simulink library "trot_Gait"  (R2024a)
settings: Solver=VariableStepAuto  StartTime=0.0  StopTime=10.0  RelTol=1e-3
undefined symbols (not defined in the file): Lower_limbs, P0x, P0z, P1x, P1z, P2x, P2z, P3x, P3z, Upper_limbs
libraries: Plane_Movement_trot_forward x4
settings Model: Creator=renre  LastModifiedBy=renre

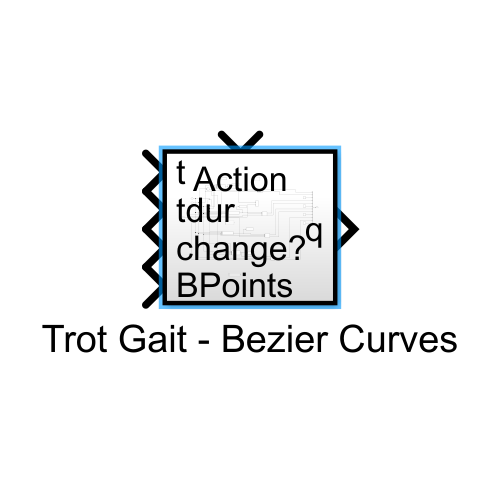
[thumbnail: Simulink's stored preview of the top-level diagram]
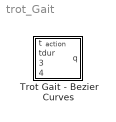
== system trot_Gait ==
  Trot Gait - Bezier Curves : Subsystem

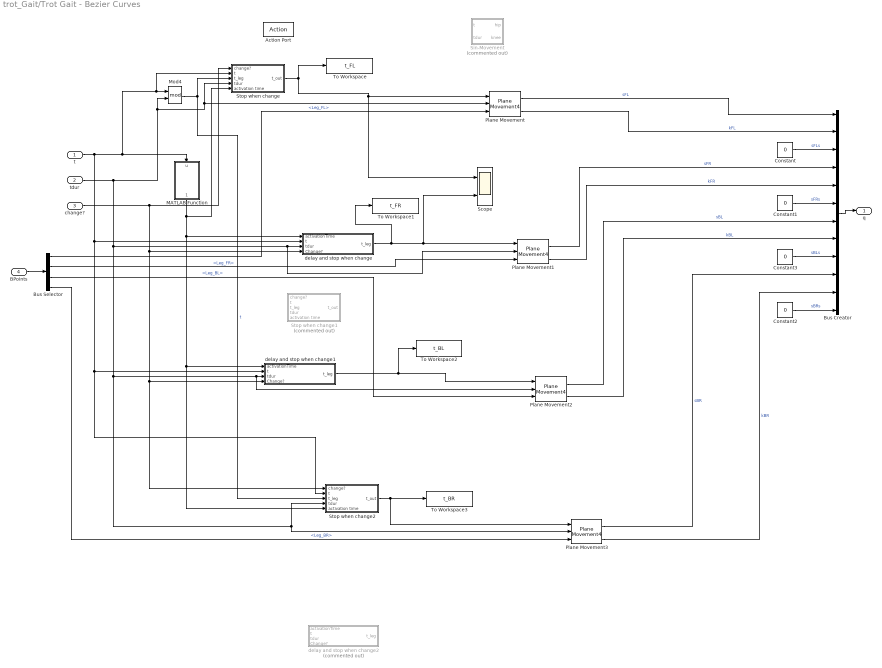
== system trot_Gait/Trot Gait - Bezier Curves ==
  t : Inport
  tdur : Inport  Port=2
  change? : Inport  Port=3
  BPoints : Inport  Port=4
  Action Port : ActionPort  InitializeStates=reset
  Bus Creator : BusCreator  Inputs=12
  Bus Selector : BusSelector  OutputSignals=Leg_FL,Leg_FR,Leg_BL,Leg_BR
  Constant{,1..3} (4 alike) : Constant  Value=0
  MATLAB Function : MATLAB Function  TreatAsAtomicUnit=on
  Mod4 : Math  Operator=mod
  Plane Movement{,1..3} (4 alike) : Plane_Movement_trot_forward/Plane Movement4  SystemSampleTime=-1  VariantActivationTime=update diagram  AllowFlexibleInterface=on  Latency=0  AutoFrameSizeCalculation=off
  Scope : Scope  NumInputPorts=2
  Sin-Movement : Subsystem  Commented=on
  Stop when change : Subsystem
  Stop when change1 : Subsystem  Commented=on
  Stop when change2 : Subsystem
  To Workspace : ToWorkspace  VariableName=t_FL  SaveFormat=Structure With Time  SampleTime=-1
  To Workspace1 : ToWorkspace  VariableName=t_FR  SaveFormat=Structure  SampleTime=-1
  To Workspace2 : ToWorkspace  VariableName=t_BL  SaveFormat=Structure  SampleTime=-1
  To Workspace3 : ToWorkspace  VariableName=t_BR  SaveFormat=Structure  SampleTime=-1
  delay and stop when change : Subsystem  mask{delay=0.5}
  delay and stop when change1 : Subsystem  mask{delay=0.5}
  delay and stop when change2 : Subsystem  Commented=on  mask{delay=0}
  q : Outport
  wires:
  BPoints/1 -> Bus Selector/1
  Stop when change/1(t_out) -> To Workspace/1, Plane Movement/1, Scope/1
  Stop when change2/1(t_out) -> Plane Movement3/1, To Workspace3/1
  delay and stop when change1/1(t_leg) -> Plane Movement2/1, To Workspace2/1
  delay and stop when change/1(t_leg) -> Plane Movement1/1, Scope/2, To Workspace1/1
  MATLAB Function/1(activationTime) -> delay and stop when change/1(activationTime), delay and stop when change1/1(activationTime), Stop when change2/5(activation time), Stop when change/5(activation time)
  change?/1 -> delay and stop when change/4(Change?), delay and stop when change1/4(Change?), Stop when change2/1(change?), Stop when change/1(change?)
  Constant2/1 -> Bus Creator/12  "sBRs"
  Constant3/1 -> Bus Creator/9  "sBLs"
  Constant1/1 -> Bus Creator/6  "sFRs"
  Constant/1 -> Bus Creator/3  "sFLs"
  Mod4/1 -> Stop when change/3(t_leg), Stop when change2/3(t_leg)  "t"
  tdur/1 -> delay and stop when change1/3(tdur), Plane Movement2/2, Plane Movement3/2, Stop when change2/4(tdur), delay and stop when change/3(tdur), Plane Movement1/2, Mod4/2, Plane Movement/2, Stop when change/4(tdur)
  t/1 -> Mod4/1, Stop when change/2(t), MATLAB Function/1(u), delay and stop when change/2(t), delay and stop when change1/2(t), Stop when change2/2(t)
  Plane Movement3/1 -> Bus Creator/10  "sBR"
  Plane Movement3/2 -> Bus Creator/11  "kBR"
  Plane Movement2/1 -> Bus Creator/7  "sBL"
  Plane Movement2/2 -> Bus Creator/8  "kBL"
  Plane Movement1/2 -> Bus Creator/5  "kFR"
  Plane Movement/2 -> Bus Creator/2  "kFL"
  Plane Movement1/1 -> Bus Creator/4  "sFR"
  Plane Movement/1 -> Bus Creator/1  "sFL"
  Bus Creator/1 -> q/1
  Bus Selector/1 -> Plane Movement/3  "<Leg_FL>"
  Bus Selector/2 -> Plane Movement1/3  "<Leg_FR>"
  Bus Selector/3 -> Plane Movement2/3  "<Leg_BL>"
  Bus Selector/4 -> Plane Movement3/3  "<Leg_BR>"

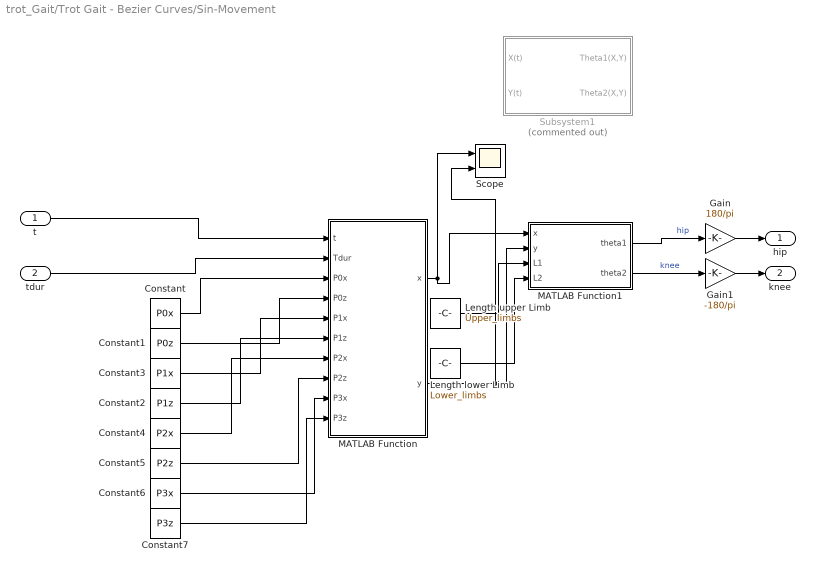
== system trot_Gait/Trot Gait - Bezier Curves/Sin-Movement ==
  t : Inport
  tdur : Inport  Port=2
  Constant : Constant  Value=P0x
  Constant1 : Constant  Value=P0z
  Constant2 : Constant  Value=P1z
  Constant3 : Constant  Value=P1x
  Constant4 : Constant  Value=P2x
  Constant5 : Constant  Value=P2z
  Constant6 : Constant  Value=P3x
  Constant7 : Constant  Value=P3z
  Gain : Gain  Gain=180/pi
  Gain1 : Gain  Gain=-180/pi
  Length lower Limb : Constant  Value=Lower_limbs
  Length upper Limb : Constant  Value=Upper_limbs
  MATLAB Function : MATLAB Function  TreatAsAtomicUnit=on
  MATLAB Function1 : MATLAB Function  TreatAsAtomicUnit=on
  Scope : Scope  NumInputPorts=2
  Subsystem1 : Subsystem  Commented=on
  hip : Outport
  knee : Outport  Port=2
  wires:
  Constant7/1 -> MATLAB Function/10(P3z)
  Constant6/1 -> MATLAB Function/9(P3x)
  Constant5/1 -> MATLAB Function/8(P2z)
  Constant4/1 -> MATLAB Function/7(P2x)
  Constant2/1 -> MATLAB Function/6(P1z)
  Constant3/1 -> MATLAB Function/5(P1x)
  Constant1/1 -> MATLAB Function/4(P0z)
  Constant/1 -> MATLAB Function/3(P0x)
  Gain/1 -> hip/1
  Gain1/1 -> knee/1
  Length lower Limb/1 -> MATLAB Function1/4(L2)
  Length upper Limb/1 -> MATLAB Function1/3(L1)
  t/1 -> MATLAB Function/1(t)
  MATLAB Function1/1(theta1) -> Gain/1  "hip"
  tdur/1 -> MATLAB Function/2(Tdur)
  MATLAB Function1/2(theta2) -> Gain1/1  "knee"
  MATLAB Function/1(x) -> Scope/1, MATLAB Function1/1(x)
  MATLAB Function/2(y) -> Scope/2, MATLAB Function1/2(y)

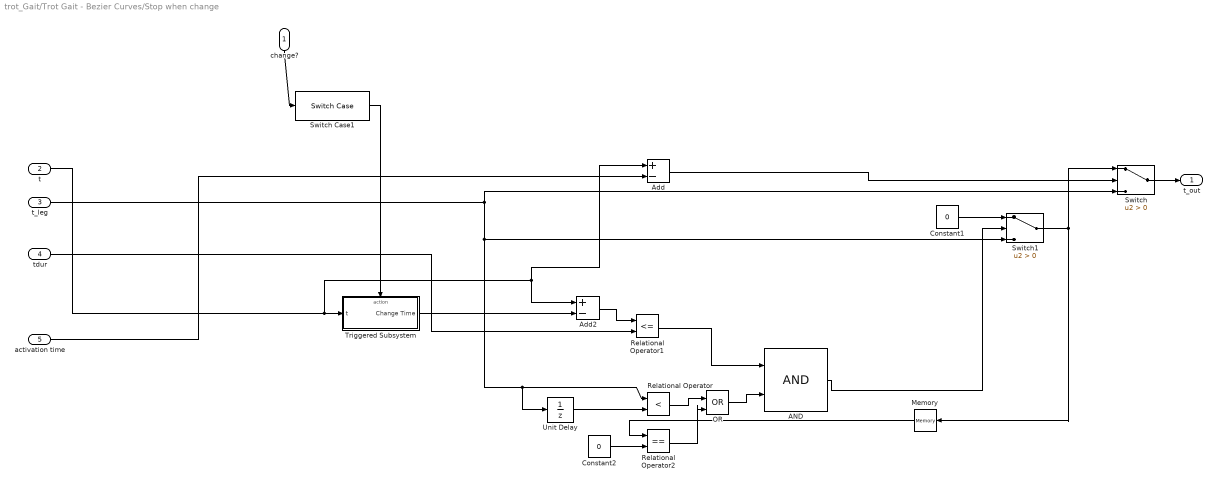
== system trot_Gait/Trot Gait - Bezier Curves/Stop when change ==
  change? : Inport
  t : Inport  Port=2
  t_leg : Inport  Port=3
  tdur : Inport  Port=4
  activation time : Inport  Port=5
  AND : Logic  IconShape=distinctive  AllPortsSameDT=off  OutDataTypeStr=boolean
  Add : Sum  Inputs=+-
  Add2 : Sum  Inputs=+-
  Constant1 : Constant  Value=0
  Constant2 : Constant  Value=0
  Memory : Memory
  OR : Logic  Operator=OR  IconShape=distinctive  AllPortsSameDT=off  OutDataTypeStr=boolean
  Relational Operator : RelationalOperator  Operator=<  OutDataTypeStr=boolean  RndMeth=Simplest  InputSameDT=off
  Relational Operator1 : RelationalOperator  Operator=<=  OutDataTypeStr=boolean  RndMeth=Simplest  InputSameDT=off
  Relational Operator2 : RelationalOperator  Operator===  OutDataTypeStr=boolean  RndMeth=Simplest  InputSameDT=off
  Switch : Switch  Criteria=u2 > Threshold  SaturateOnIntegerOverflow=off  InputSameDT=off
  Switch Case1 : SwitchCase  ShowDefaultCase=off
  Switch1 : Switch  Criteria=u2 > Threshold  SaturateOnIntegerOverflow=off  InputSameDT=off
  Triggered Subsystem : Subsystem  TreatAsAtomicUnit=on
  Unit Delay : UnitDelay  SampleTime=-1  HasFrameUpgradeWarning=on
  t_out : Outport
  wires:
  Memory/1 -> Relational Operator2/1
  activation time/1 -> Add/2
  Switch/1 -> t_out/1
  Add/1 -> Switch/2
  t/1 -> Triggered Subsystem/1(t), Add/1, Add2/1
  Constant1/1 -> Switch1/1
  OR/1 -> AND/2
  Relational Operator2/1 -> OR/2
  tdur/1 -> Relational Operator1/2
  Relational Operator/1 -> OR/1
  Triggered Subsystem/1(Change Time) -> Add2/2
  Constant2/1 -> Relational Operator2/2
  Relational Operator1/1 -> AND/1
  Switch1/1 -> Switch/1, Memory/1
  Unit Delay/1 -> Relational Operator/2
  AND/1 -> Switch1/2
  Switch Case1/1 -> Triggered Subsystem/Action
  change?/1 -> Switch Case1/1
  Add2/1 -> Relational Operator1/1
  t_leg/1 -> Relational Operator/1, Unit Delay/1, Switch1/3, Switch/3

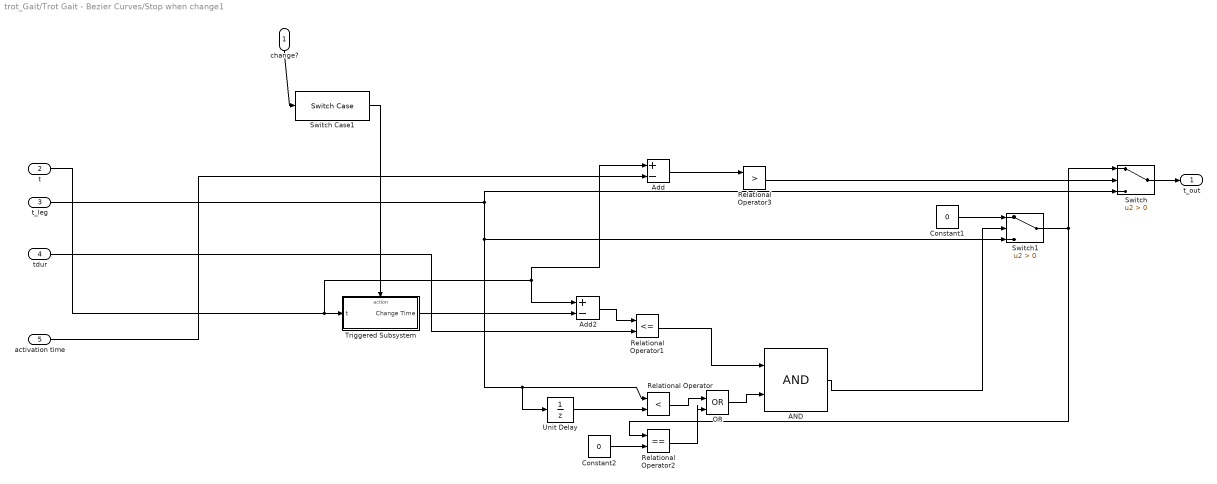
== system trot_Gait/Trot Gait - Bezier Curves/Stop when change1 ==
  change? : Inport
  t : Inport  Port=2
  t_leg : Inport  Port=3
  tdur : Inport  Port=4
  activation time : Inport  Port=5
  AND : Logic  IconShape=distinctive  AllPortsSameDT=off  OutDataTypeStr=boolean
  Add : Sum  Inputs=+-
  Add2 : Sum  Inputs=+-
  Constant1 : Constant  Value=0
  Constant2 : Constant  Value=0
  OR : Logic  Operator=OR  IconShape=distinctive  AllPortsSameDT=off  OutDataTypeStr=boolean
  Relational Operator : RelationalOperator  Operator=<  OutDataTypeStr=boolean  RndMeth=Simplest  InputSameDT=off
  Relational Operator1 : RelationalOperator  Operator=<=  OutDataTypeStr=boolean  RndMeth=Simplest  InputSameDT=off
  Relational Operator2 : RelationalOperator  Operator===  OutDataTypeStr=boolean  RndMeth=Simplest  InputSameDT=off
  Relational Operator3 : RelationalOperator  Operator=>  OutDataTypeStr=boolean  RndMeth=Simplest  InputSameDT=off
  Switch : Switch  Criteria=u2 > Threshold  SaturateOnIntegerOverflow=off  InputSameDT=off
  Switch Case1 : SwitchCase  ShowDefaultCase=off
  Switch1 : Switch  Criteria=u2 > Threshold  SaturateOnIntegerOverflow=off  InputSameDT=off
  Triggered Subsystem : Subsystem  TreatAsAtomicUnit=on
  Unit Delay : UnitDelay  SampleTime=-1  HasFrameUpgradeWarning=on
  t_out : Outport
  wires:
  t_leg/1 -> Switch/3, Switch1/3, Unit Delay/1, Relational Operator/1
  Add2/1 -> Relational Operator1/1
  change?/1 -> Switch Case1/1
  Switch Case1/1 -> Triggered Subsystem/Action
  AND/1 -> Switch1/2
  Unit Delay/1 -> Relational Operator/2
  Switch1/1 -> Relational Operator2/1, Switch/1
  Relational Operator1/1 -> AND/1
  Constant2/1 -> Relational Operator2/2
  Triggered Subsystem/1(Change Time) -> Add2/2
  Relational Operator/1 -> OR/1
  tdur/1 -> Relational Operator1/2
  Relational Operator2/1 -> OR/2
  OR/1 -> AND/2
  Constant1/1 -> Switch1/1
  t/1 -> Add2/1, Add/1, Triggered Subsystem/1(t)
  Relational Operator3/1 -> Switch/2
  Switch/1 -> t_out/1
  Add/1 -> Relational Operator3/1
  activation time/1 -> Add/2

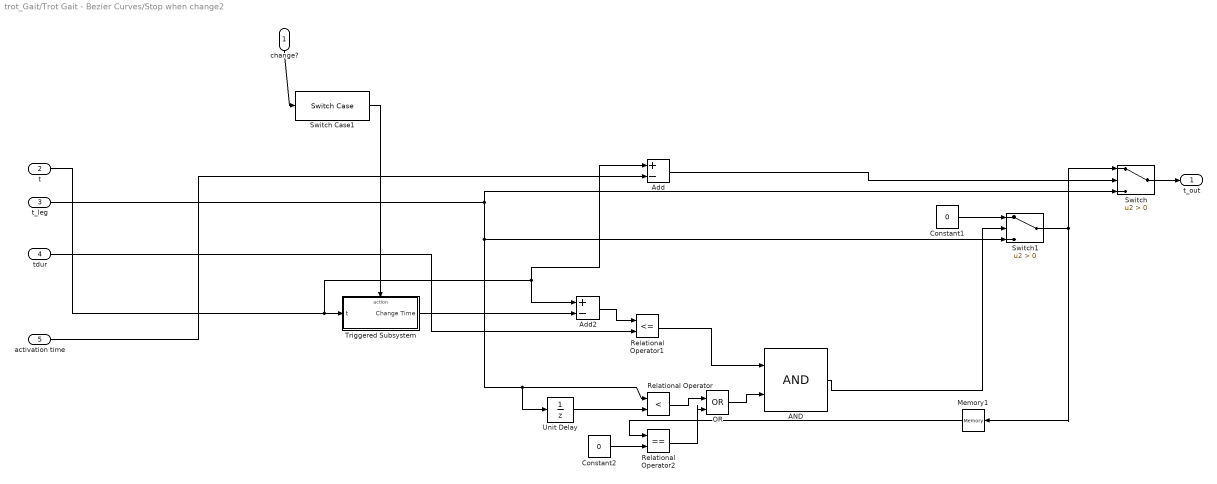
== system trot_Gait/Trot Gait - Bezier Curves/Stop when change2 ==
  change? : Inport
  t : Inport  Port=2
  t_leg : Inport  Port=3
  tdur : Inport  Port=4
  activation time : Inport  Port=5
  AND : Logic  IconShape=distinctive  AllPortsSameDT=off  OutDataTypeStr=boolean
  Add : Sum  Inputs=+-
  Add2 : Sum  Inputs=+-
  Constant1 : Constant  Value=0
  Constant2 : Constant  Value=0
  Memory1 : Memory
  OR : Logic  Operator=OR  IconShape=distinctive  AllPortsSameDT=off  OutDataTypeStr=boolean
  Relational Operator : RelationalOperator  Operator=<  OutDataTypeStr=boolean  RndMeth=Simplest  InputSameDT=off
  Relational Operator1 : RelationalOperator  Operator=<=  OutDataTypeStr=boolean  RndMeth=Simplest  InputSameDT=off
  Relational Operator2 : RelationalOperator  Operator===  OutDataTypeStr=boolean  RndMeth=Simplest  InputSameDT=off
  Switch : Switch  Criteria=u2 > Threshold  SaturateOnIntegerOverflow=off  InputSameDT=off
  Switch Case1 : SwitchCase  ShowDefaultCase=off
  Switch1 : Switch  Criteria=u2 > Threshold  SaturateOnIntegerOverflow=off  InputSameDT=off
  Triggered Subsystem : Subsystem  TreatAsAtomicUnit=on
  Unit Delay : UnitDelay  SampleTime=-1  HasFrameUpgradeWarning=on
  t_out : Outport
  wires:
  Memory1/1 -> Relational Operator2/1
  activation time/1 -> Add/2
  Switch/1 -> t_out/1
  Add/1 -> Switch/2
  t/1 -> Triggered Subsystem/1(t), Add/1, Add2/1
  Constant1/1 -> Switch1/1
  OR/1 -> AND/2
  Relational Operator2/1 -> OR/2
  tdur/1 -> Relational Operator1/2
  Relational Operator/1 -> OR/1
  Triggered Subsystem/1(Change Time) -> Add2/2
  Constant2/1 -> Relational Operator2/2
  Relational Operator1/1 -> AND/1
  Switch1/1 -> Switch/1, Memory1/1
  Unit Delay/1 -> Relational Operator/2
  AND/1 -> Switch1/2
  Switch Case1/1 -> Triggered Subsystem/Action
  change?/1 -> Switch Case1/1
  Add2/1 -> Relational Operator1/1
  t_leg/1 -> Relational Operator/1, Unit Delay/1, Switch1/3, Switch/3

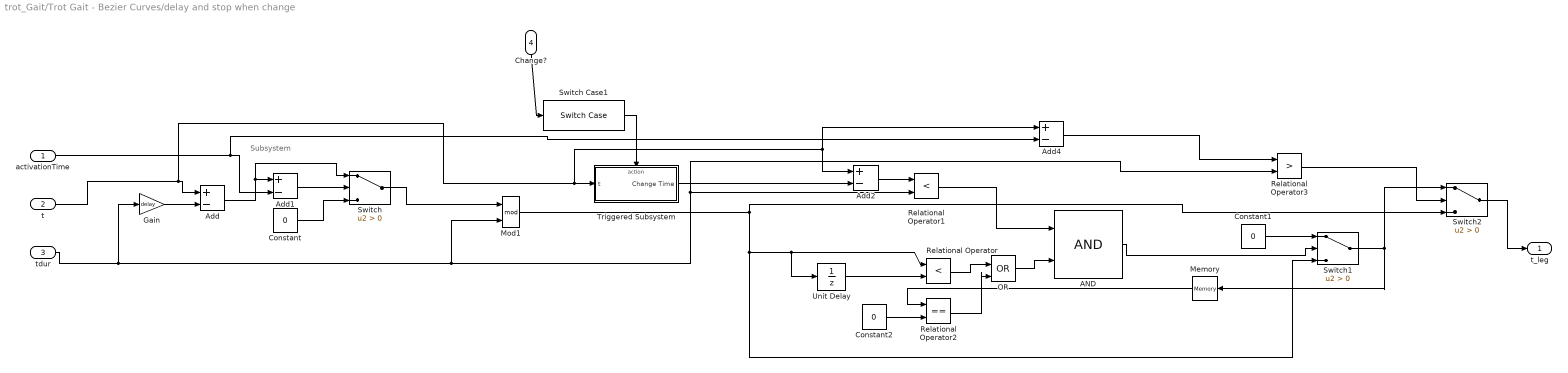
== system trot_Gait/Trot Gait - Bezier Curves/delay and stop when change ==
  note: Subsystem
  activationTime : Inport
  t : Inport  Port=2
  tdur : Inport  Port=3
  Change? : Inport  Port=4
  AND : Logic  IconShape=distinctive  AllPortsSameDT=off  OutDataTypeStr=boolean
  Add{,1..2,4} (4 alike) : Sum  Inputs=+-
  Constant : Constant  Value=0
  Constant1 : Constant  Value=0
  Constant2 : Constant  Value=0
  Gain : Gain  Gain=delay
  Memory : Memory
  Mod1 : Math  Operator=mod
  OR : Logic  Operator=OR  IconShape=distinctive  AllPortsSameDT=off  OutDataTypeStr=boolean
  Relational Operator : RelationalOperator  Operator=<  OutDataTypeStr=boolean  RndMeth=Simplest  InputSameDT=off
  Relational Operator1 : RelationalOperator  Operator=<  OutDataTypeStr=boolean  RndMeth=Simplest  InputSameDT=off
  Relational Operator2 : RelationalOperator  Operator===  OutDataTypeStr=boolean  RndMeth=Simplest  InputSameDT=off
  Relational Operator3 : RelationalOperator  Operator=>  OutDataTypeStr=boolean  RndMeth=Simplest  InputSameDT=off
  Switch : Switch  Criteria=u2 > Threshold  SaturateOnIntegerOverflow=off  InputSameDT=off
  Switch Case1 : SwitchCase  ShowDefaultCase=off
  Switch1 : Switch  Criteria=u2 > Threshold  SaturateOnIntegerOverflow=off  InputSameDT=off
  Switch2 : Switch  Criteria=u2 > Threshold  SaturateOnIntegerOverflow=off  InputSameDT=off
  Triggered Subsystem : Subsystem  TreatAsAtomicUnit=on
  Unit Delay : UnitDelay  SampleTime=-1  HasFrameUpgradeWarning=on
  t_leg : Outport
  wires:
  Memory/1 -> Relational Operator2/1
  Add4/1 -> Relational Operator3/1
  tdur/1 -> Relational Operator1/2, Relational Operator3/2, Mod1/2, Gain/1
  Relational Operator3/1 -> Switch2/2
  Switch2/1 -> t_leg/1
  OR/1 -> AND/2
  Constant2/1 -> Relational Operator2/2
  Relational Operator2/1 -> OR/2
  Add2/1 -> Relational Operator1/1
  Triggered Subsystem/1(Change Time) -> Add2/2
  Mod1/1 -> Relational Operator/1, Unit Delay/1, Switch1/3, Switch2/3
  Switch1/1 -> Memory/1, Switch2/1
  AND/1 -> Switch1/2
  Unit Delay/1 -> Relational Operator/2
  Change?/1 -> Switch Case1/1
  Relational Operator/1 -> OR/1
  Constant1/1 -> Switch1/1
  Relational Operator1/1 -> AND/1
  Switch Case1/1 -> Triggered Subsystem/Action
  Add/1 -> Add1/1, Switch/1
  activationTime/1 -> Add1/2, Add4/2
  Add1/1 -> Switch/2
  Constant/1 -> Switch/3
  t/1 -> Add/1, Triggered Subsystem/1(t), Add4/1, Add2/1
  Gain/1 -> Add/2
  Switch/1 -> Mod1/1

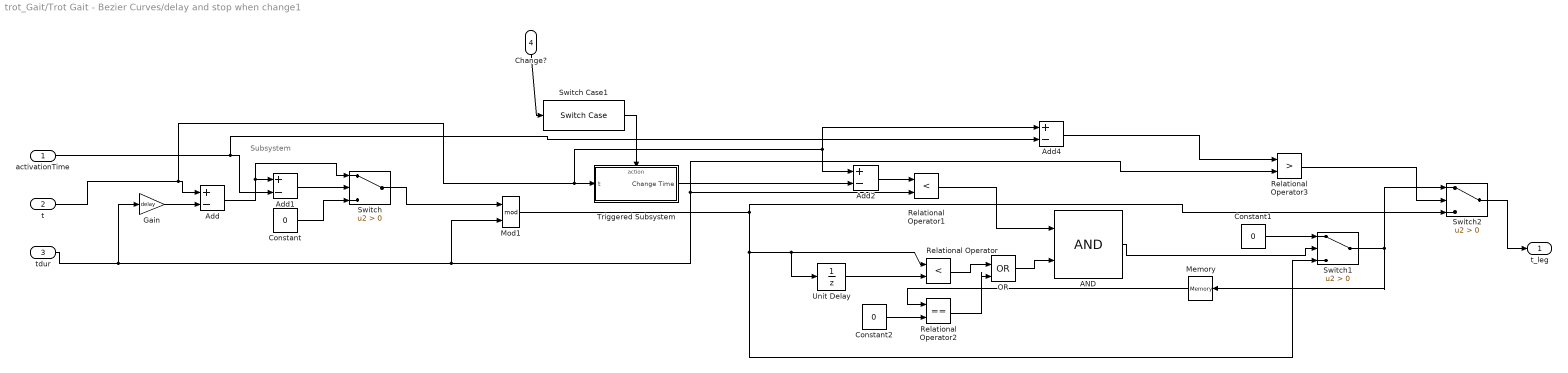
== system trot_Gait/Trot Gait - Bezier Curves/delay and stop when change1 ==
  note: Subsystem
  activationTime : Inport
  t : Inport  Port=2
  tdur : Inport  Port=3
  Change? : Inport  Port=4
  AND : Logic  IconShape=distinctive  AllPortsSameDT=off  OutDataTypeStr=boolean
  Add{,1..2,4} (4 alike) : Sum  Inputs=+-
  Constant : Constant  Value=0
  Constant1 : Constant  Value=0
  Constant2 : Constant  Value=0
  Gain : Gain  Gain=delay
  Memory : Memory
  Mod1 : Math  Operator=mod
  OR : Logic  Operator=OR  IconShape=distinctive  AllPortsSameDT=off  OutDataTypeStr=boolean
  Relational Operator : RelationalOperator  Operator=<  OutDataTypeStr=boolean  RndMeth=Simplest  InputSameDT=off
  Relational Operator1 : RelationalOperator  Operator=<  OutDataTypeStr=boolean  RndMeth=Simplest  InputSameDT=off
  Relational Operator2 : RelationalOperator  Operator===  OutDataTypeStr=boolean  RndMeth=Simplest  InputSameDT=off
  Relational Operator3 : RelationalOperator  Operator=>  OutDataTypeStr=boolean  RndMeth=Simplest  InputSameDT=off
  Switch : Switch  Criteria=u2 > Threshold  SaturateOnIntegerOverflow=off  InputSameDT=off
  Switch Case1 : SwitchCase  ShowDefaultCase=off
  Switch1 : Switch  Criteria=u2 > Threshold  SaturateOnIntegerOverflow=off  InputSameDT=off
  Switch2 : Switch  Criteria=u2 > Threshold  SaturateOnIntegerOverflow=off  InputSameDT=off
  Triggered Subsystem : Subsystem  TreatAsAtomicUnit=on
  Unit Delay : UnitDelay  SampleTime=-1  HasFrameUpgradeWarning=on
  t_leg : Outport
  wires:
  Memory/1 -> Relational Operator2/1
  Add4/1 -> Relational Operator3/1
  tdur/1 -> Relational Operator1/2, Relational Operator3/2, Mod1/2, Gain/1
  Relational Operator3/1 -> Switch2/2
  Switch2/1 -> t_leg/1
  OR/1 -> AND/2
  Constant2/1 -> Relational Operator2/2
  Relational Operator2/1 -> OR/2
  Add2/1 -> Relational Operator1/1
  Triggered Subsystem/1(Change Time) -> Add2/2
  Mod1/1 -> Relational Operator/1, Unit Delay/1, Switch1/3, Switch2/3
  Switch1/1 -> Memory/1, Switch2/1
  AND/1 -> Switch1/2
  Unit Delay/1 -> Relational Operator/2
  Change?/1 -> Switch Case1/1
  Relational Operator/1 -> OR/1
  Constant1/1 -> Switch1/1
  Relational Operator1/1 -> AND/1
  Switch Case1/1 -> Triggered Subsystem/Action
  Add/1 -> Add1/1, Switch/1
  activationTime/1 -> Add1/2, Add4/2
  Add1/1 -> Switch/2
  Constant/1 -> Switch/3
  t/1 -> Add/1, Triggered Subsystem/1(t), Add4/1, Add2/1
  Gain/1 -> Add/2
  Switch/1 -> Mod1/1

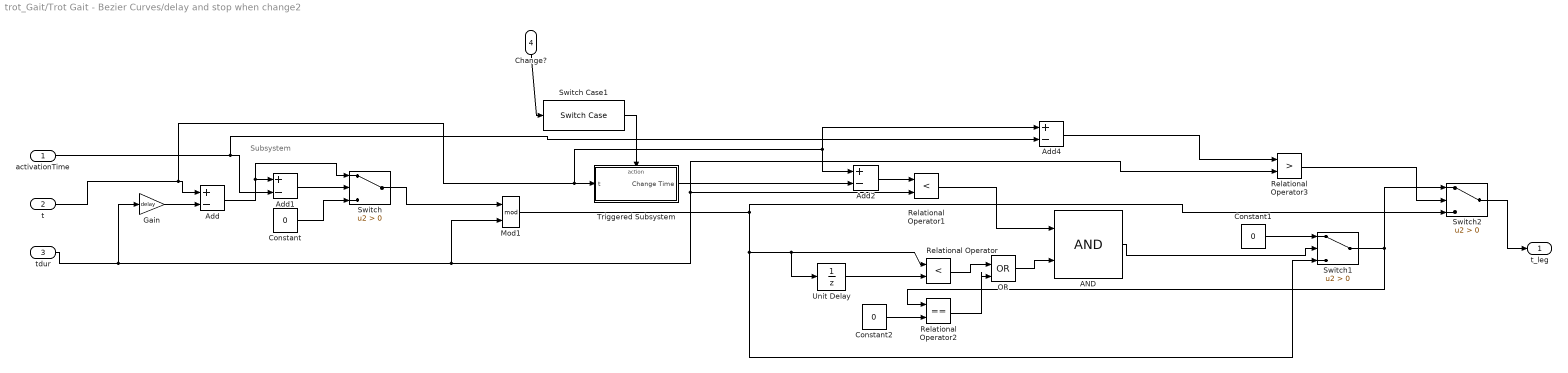
== system trot_Gait/Trot Gait - Bezier Curves/delay and stop when change2 ==
  note: Subsystem
  activationTime : Inport
  t : Inport  Port=2
  tdur : Inport  Port=3
  Change? : Inport  Port=4
  AND : Logic  IconShape=distinctive  AllPortsSameDT=off  OutDataTypeStr=boolean
  Add{,1..2,4} (4 alike) : Sum  Inputs=+-
  Constant : Constant  Value=0
  Constant1 : Constant  Value=0
  Constant2 : Constant  Value=0
  Gain : Gain  Gain=delay
  Mod1 : Math  Operator=mod
  OR : Logic  Operator=OR  IconShape=distinctive  AllPortsSameDT=off  OutDataTypeStr=boolean
  Relational Operator : RelationalOperator  Operator=<  OutDataTypeStr=boolean  RndMeth=Simplest  InputSameDT=off
  Relational Operator1 : RelationalOperator  Operator=<  OutDataTypeStr=boolean  RndMeth=Simplest  InputSameDT=off
  Relational Operator2 : RelationalOperator  Operator===  OutDataTypeStr=boolean  RndMeth=Simplest  InputSameDT=off
  Relational Operator3 : RelationalOperator  Operator=>  OutDataTypeStr=boolean  RndMeth=Simplest  InputSameDT=off
  Switch : Switch  Criteria=u2 > Threshold  SaturateOnIntegerOverflow=off  InputSameDT=off
  Switch Case1 : SwitchCase  ShowDefaultCase=off
  Switch1 : Switch  Criteria=u2 > Threshold  SaturateOnIntegerOverflow=off  InputSameDT=off
  Switch2 : Switch  Criteria=u2 > Threshold  SaturateOnIntegerOverflow=off  InputSameDT=off
  Triggered Subsystem : Subsystem  TreatAsAtomicUnit=on
  Unit Delay : UnitDelay  SampleTime=-1  HasFrameUpgradeWarning=on
  t_leg : Outport
  wires:
  Add4/1 -> Relational Operator3/1
  tdur/1 -> Relational Operator1/2, Relational Operator3/2, Mod1/2, Gain/1
  Relational Operator3/1 -> Switch2/2
  Switch2/1 -> t_leg/1
  OR/1 -> AND/2
  Constant2/1 -> Relational Operator2/2
  Relational Operator2/1 -> OR/2
  Add2/1 -> Relational Operator1/1
  Triggered Subsystem/1(Change Time) -> Add2/2
  Mod1/1 -> Relational Operator/1, Unit Delay/1, Switch1/3, Switch2/3
  Switch1/1 -> Relational Operator2/1, Switch2/1
  AND/1 -> Switch1/2
  Unit Delay/1 -> Relational Operator/2
  Change?/1 -> Switch Case1/1
  Relational Operator/1 -> OR/1
  Constant1/1 -> Switch1/1
  Relational Operator1/1 -> AND/1
  Switch Case1/1 -> Triggered Subsystem/Action
  Add/1 -> Add1/1, Switch/1
  activationTime/1 -> Add1/2, Add4/2
  Add1/1 -> Switch/2
  Constant/1 -> Switch/3
  t/1 -> Add/1, Triggered Subsystem/1(t), Add4/1, Add2/1
  Gain/1 -> Add/2
  Switch/1 -> Mod1/1

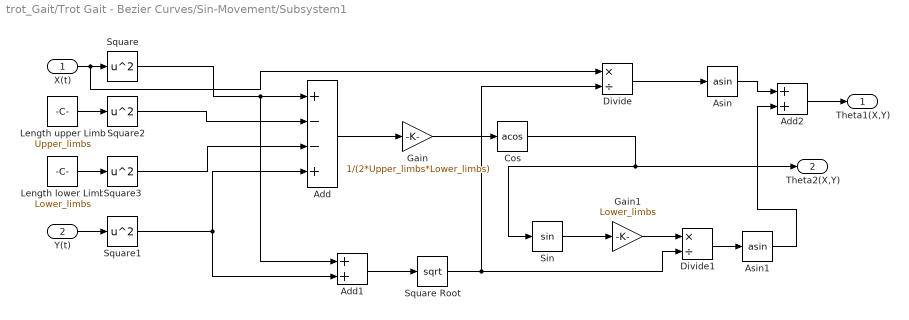
== system trot_Gait/Trot Gait - Bezier Curves/Sin-Movement/Subsystem1 ==
  X(t) : Inport
  Y(t) : Inport  Port=2
  Add : Sum  Inputs=+--+
  Add1 : Sum
  Add2 : Sum
  Asin : Trigonometry  Operator=asin
  Asin1 : Trigonometry  Operator=asin
  Cos : Trigonometry  Operator=acos
  Divide : Product  Inputs=*/
  Divide1 : Product  Inputs=*/
  Gain : Gain  Gain=1/(2*Upper_limbs*Lower_limbs)
  Gain1 : Gain  Gain=Lower_limbs
  Length lower Limb : Constant  Value=Lower_limbs
  Length upper Limb : Constant  Value=Upper_limbs
  Sin : Trigonometry
  Square{,1..3} (4 alike) : Math  Operator=square
  Square Root : Sqrt
  Theta1(X,Y) : Outport
  Theta2(X,Y) : Outport  Port=2
  wires:
  Divide/1 -> Asin/1
  Add2/1 -> Theta1(X,Y)/1
  Asin1/1 -> Add2/2
  Divide1/1 -> Asin1/1
  Square Root/1 -> Divide1/2, Divide/2
  Gain1/1 -> Divide1/1
  Add1/1 -> Square Root/1
  Sin/1 -> Gain1/1
  Asin/1 -> Add2/1
  Cos/1 -> Sin/1, Theta2(X,Y)/1
  Gain/1 -> Cos/1
  Add/1 -> Gain/1
  Square1/1 -> Add/4, Add1/2
  Square3/1 -> Add/3
  Square2/1 -> Add/2
  Length lower Limb/1 -> Square3/1
  Length upper Limb/1 -> Square2/1
  Square/1 -> Add/1, Add1/1
  Y(t)/1 -> Square1/1
  X(t)/1 -> Square/1, Divide/1

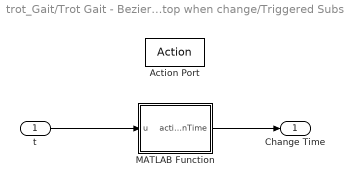
== system trot_Gait/Trot Gait - Bezier Curves/Stop when change/Triggered Subsystem ==
  t : Inport
  Action Port : ActionPort  InitializeStates=reset
  MATLAB Function : MATLAB Function  TreatAsAtomicUnit=on
  Change Time : Outport
  wires:
  t/1 -> MATLAB Function/1(u)
  MATLAB Function/1(activationTime) -> Change Time/1

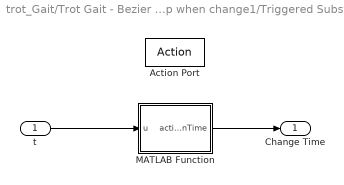
== system trot_Gait/Trot Gait - Bezier Curves/Stop when change1/Triggered Subsystem ==
  t : Inport
  Action Port : ActionPort  InitializeStates=reset
  MATLAB Function : MATLAB Function  TreatAsAtomicUnit=on
  Change Time : Outport
  wires:
  MATLAB Function/1(activationTime) -> Change Time/1
  t/1 -> MATLAB Function/1(u)

== system trot_Gait/Trot Gait - Bezier Curves/Stop when change2/Triggered Subsystem ==
  t : Inport
  Action Port : ActionPort  InitializeStates=reset
  MATLAB Function : MATLAB Function  TreatAsAtomicUnit=on
  Change Time : Outport
  wires:
  t/1 -> MATLAB Function/1(u)
  MATLAB Function/1(activationTime) -> Change Time/1

== system trot_Gait/Trot Gait - Bezier Curves/delay and stop when change/Triggered Subsystem ==
  t : Inport
  Action Port : ActionPort  InitializeStates=reset
  MATLAB Function : MATLAB Function  TreatAsAtomicUnit=on
  Change Time : Outport
  wires:
  t/1 -> MATLAB Function/1(u)
  MATLAB Function/1(activationTime) -> Change Time/1

== system trot_Gait/Trot Gait - Bezier Curves/delay and stop when change1/Triggered Subsystem ==
  t : Inport
  Action Port : ActionPort  InitializeStates=reset
  MATLAB Function : MATLAB Function  TreatAsAtomicUnit=on
  Change Time : Outport
  wires:
  t/1 -> MATLAB Function/1(u)
  MATLAB Function/1(activationTime) -> Change Time/1

== system trot_Gait/Trot Gait - Bezier Curves/delay and stop when change2/Triggered Subsystem ==
  t : Inport
  Action Port : ActionPort  InitializeStates=reset
  MATLAB Function : MATLAB Function  TreatAsAtomicUnit=on
  Change Time : Outport
  wires:
  t/1 -> MATLAB Function/1(u)
  MATLAB Function/1(activationTime) -> Change Time/1

== matlab function trot_Gait/Trot Gait - Bezier Curves/Sin-Movement/MATLAB Function ==
  data: x output; t input; y output; Tdur input; P0x input; P0z input; P1x input; P1z input; P2x input; P2z input; P3x input; P3z input
function [x, y] = bezTrajV2(t, Tdur, P0x,P0z,P1x,P1z,P2x,P2z,P3x,P3z)
t_swing = Tdur/4;
t_support = Tdur*3/4;

P0 = [P0x, P0z];
P1 = [P1x, P1z];
P2 = [P2x, P2z];
P3 = [P3x, P3z];
if t<=t_swing
    Sw = P0*((1-(t/t_swing))^3) + 3*P1*(t/t_swing)*((1-(t/t_swing))^2) + 3*P2*((t/t_swing)^2)*(1-(t/t_swing)) + P3*((t/t_swing)^3);
    
    x = -1*Sw(1);
    y = Sw(2);
else
    x = -1*(P3(1)+(P0(1)-P3(1))/t_support*(t-t_swing));
    y = -0.003*sin((x-P0(1))*pi/(P3(1)-P0(1)))+P0(2);
end
end

== matlab function trot_Gait/Trot Gait - Bezier Curves/Sin-Movement/MATLAB Function1 ==
  data: x input; theta1 output; y input; L1 input; L2 input; theta2 output
function [theta1, theta2] = ang(x,y,L1,L2)
theta2 = acos((x.^2+y.^2-L1.^2-L2.^2) / (2*L1*L2));
beta = asin((L2*sin(theta2))./((x.^2+y.^2).^0.5));
theta1 = asin(x./((x.^2+y.^2).^0.5)) + beta;
end

== matlab function trot_Gait/Trot Gait - Bezier Curves/Stop when change1/Triggered Subsystem/MATLAB Function ==
  data: u input; activationTime output
function activationTime = getActivationTime(u)
    persistent t_start
    if isempty(t_start)
        t_start = u;
    end
    activationTime = t_start;
end

== matlab function trot_Gait/Trot Gait - Bezier Curves/Stop when change2/Triggered Subsystem/MATLAB Function ==
  data: u input; activationTime output
function activationTime = getActivationTime(u)
    persistent t_start
    if isempty(t_start)
        t_start = u;
    end
    activationTime = t_start;
end

== matlab function trot_Gait/Trot Gait - Bezier Curves/MATLAB Function ==
  data: u input; activationTime output
function activationTime = getActivationTime(u)
    persistent t_start
    if isempty(t_start)
        t_start = u;
    end
    activationTime = t_start;
end

== matlab function trot_Gait/Trot Gait - Bezier Curves/Stop when change/Triggered Subsystem/MATLAB Function ==
  data: u input; activationTime output
function activationTime = getActivationTime(u)
    persistent t_start
    if isempty(t_start)
        t_start = u;
    end
    activationTime = t_start;
end

== matlab function trot_Gait/Trot Gait - Bezier Curves/delay and stop when change/Triggered Subsystem/MATLAB Function ==
  data: u input; activationTime output
function activationTime = getActivationTime(u)
    persistent t_start
    if isempty(t_start)
        t_start = u;
    end
    activationTime = t_start;
end

== matlab function trot_Gait/Trot Gait - Bezier Curves/delay and stop when change1/Triggered Subsystem/MATLAB Function ==
  data: u input; activationTime output
function activationTime = getActivationTime(u)
    persistent t_start
    if isempty(t_start)
        t_start = u;
    end
    activationTime = t_start;
end

== matlab function trot_Gait/Trot Gait - Bezier Curves/delay and stop when change2/Triggered Subsystem/MATLAB Function ==
  data: u input; activationTime output
function activationTime = getActivationTime(u)
    persistent t_start
    if isempty(t_start)
        t_start = u;
    end
    activationTime = t_start;
end
